simulink model "MotDynamic"  (R2020a)
settings: Solver=VariableStepAuto  StartTime=0.0  StopTime=inf  RelTol=1e-3  EnableMultiTasking=on
model workspace (MAT data in the model file):
  EV_current = 200
  EV_motion = [20 4 0.8]
  EV_sf = 2000
  Fs = 0
  Fv = 0.0025
  Jcomp = 0.0227
  Ki = 1.25663706144
  Kisa = 346.6583
  Kp_d = 0.648424723701
  Kp_q = 1.13097335529
  Ksa = 85.4316
  Ksf = 1996.2651
  Ld = 0.000516
  Ldq = [0.000516 0.0009]
  Lq = 0.0009
  Mechanical = [0.0227 0.0025 0]
  P = 4
  PolePairs = 4
  Rs = 0.001
  T_max = 307
  T_mtpa = [0 30.6210532811 61.5690748203 93.1444955648 125.603920089 159.154914294 193.959648015 230.142548009 267.798503723 307.000007318]
  ba = 3.4029
  id_mtpa = [0 -1.69646410405 -6.64649055035 -14.4836473325 -24.7304283732 -36.9068843148 -50.593409792 -65.4508356078 -81.216288034 -97.6899955843]
  idq0 = [0 0]
  idq_limits = [-97.6904029428 235.234863652 254.71328176]
  iq_mtpa = [0 28.2505847591 56.2113714662 83.6599409941 110.471636122 136.609736594 162.096742578 186.986339268 211.343844145 235.235032823]
  lambda_pm = 0.18
  mechanical = [0.0227 0.0025 0]
  omega_init = 0
  theta_init = 0
libraries: autolibmotorctrlr x1, autolibpmsminterior x1, autolibinverter x1
settings Model: ModifiedByFormat=The MathWorks, Inc.  SimulationMode=accelerator  PauseTimes=10  Creator=The MathWorks, Inc.  LastModifiedBy=The MathWorks, Inc.
settings SolverCC: DecoupledContinuousIntegration=on
settings DataIOCC: DSMLogging=off  ReturnWorkspaceOutputs=off
settings DebuggingCC: UnderspecifiedInitializationDetection=Classic  MergeDetectMultiDrivingBlocksExec=none  ArithmeticOperatorsInVariantConditions=warning
settings ModelReferenceCC: PropagateSignalLabelsOutOfModel=off
settings SFSimCC: SimUseLocalCustomCode=off  CustomCodeUndefinedFunction=UseInterfaceOnly
settings RTWCC: RTWUseLocalCustomCode=off
settings CodeAppCC: StateflowObjectComments=on
settings GRTTargetCC: TargetLangStandard=C89/C90 (ANSI)
settings ConfigComp: CovMetricSettings=dsw  CovHtmlReporting=on  CovSaveCumulativeToWorkspaceVar=on  CovSaveSingleToWorkspaceVar=on  CovShowResultsExplorer=off  CovExternalEMLEnable=off
settings SimscapeCC: SimscapeNormalizeSystem=off  SimscapeNominalValues={1, 'bar'; 1, 'cm^3/s'; 1, 'bar*kg/s'; 1, 'kJ/kg'; 1, 'kW'; }

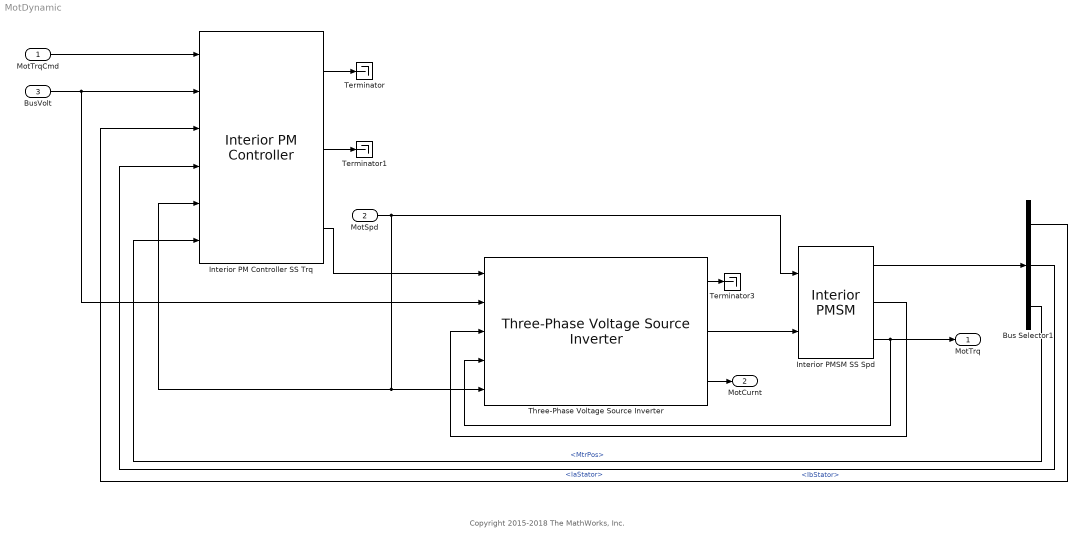
== system MotDynamic ==
  note: Copyright 2015-2018 The MathWorks, Inc.
  MotTrqCmd : Inport
  MotSpd : Inport  Port=2
  BusVolt : Inport  Port=3
  Bus Selector1 : BusSelector  OutputSignals=IaStator,IbStator,MtrPos
  Interior PM Controller SS Trq : autolibmotorctrlr/Interior PM Controller  control_type=Torque Control  Rs=Rs  Ld=Ld  Lq=Lq  lambda_pm=lambda_pm  PolePairs=PolePairs  Mechanical=Mechanical  T_max=T_max  bp=10  T_mtpa=T_mtpa  id_mtpa=id_mtpa  iq_mtpa=iq_mtpa  idq_limits=idq_limits  EV_current=EV_current  Tst=5e-5  Kp_d=Kp_d  Kp_q=Kp_q  Ki=Ki  EV_motion=EV_motion  EV_sf=EV_sf  ba=ba  Ksa=Ksa  Kisa=Kisa  Ksf=Ksf  Jcomp=Jcomp  Fv=Fv  Fs=Fs  param_loss=Single efficiency measurement  eff=98  w_loss_bp=[0 200 400 600 800 1000]  T_loss_bp=[0 25 50 75 100]  losses_table=[100 100 100 100 100;100 150 200 250 300;100 200 300 400 500;100 250 400 550 700;100 300 500 700 900;100 350 600 850 1100]  w_eff_bp=[200 400 600 800 1000]  T_eff_bp=[25 50 75 100]  efficiency_table=[96.2 98.1 98.7 99;98.1 99 99.4 99.5;98.7 99.4 99.6 99.7;99 99.5 99.7 99.8;99.2 99.6 99.7 99.8]  x_w_bp=[-1000 -800 -600 -400 -200 200 400 600 800 1000]  x_T_bp=[-100 -75 -50 -25 25 50 75 100]  x_losses_mat=[200.400801603196 225.67703109328 200.803212851408 201.612903225806 199.999999999997 200 225 200;160.320641282556 180.541624874624 201.005025125625 202.020202020203 200 200 180 160;180.541624874624 180.722891566267 181.086519114686 197.568389057748 194.999999999999 179.999999999997 180 180;201.005025125625 181.086519114686 202.020202020203 193.67991845056 190 200 179.999999999997 200;202.020202020203 197.568389057748 193.67991845056 197.505197505197 190 190 194.999999999999 200;200 194.999999999999 190 190 197.505197505197 193.67991845056 197.568389057748 202.020202020203;200 179.999999999997 200 190 193.67991845056 202.020202020203 181.086519114686 201.005025125625;180 180 179.999999999997 194.999999999999 197.568389057748 181.086519114686 180.722891566267 180.541624874624;160 180 200 200 202.020202020203 201.005025125625 180.541624874624 160.320641282556;200 225 200 199.999999999997 201.612903225806 200.803212851408 225.67703109328 200.400801603196]  Tsm=5e-4
      settings: SourceProductBaseCode=PW
  Interior PMSM SS Spd : autolibpmsminterior/Interior PMSM  port_config=Speed  sim_type=Continuous  Ts=0.001  P=P  Rs=Rs  Ldq=Ldq  KConstText=Permanent flux linkage constant (lambda_pm):  lambda_pm=lambda_pm  Ke=159.9771  mechanical=mechanical  idq0=idq0  theta_init=theta_init  omega_init=omega_init  KConst=lambda_pm  lambda_pm_calc=lambda_pm  Kt=1.323  RefBlkName='autolibpmsminterior/Interior PMSM'  aMode=1
      settings: SourceProductBaseCode=PW,MT,VE,VP
  Terminator : Terminator
  Terminator1 : Terminator
  Terminator3 : Terminator
  Three-Phase Voltage Source Inverter : autolibinverter/Three-Phase Voltage Source Inverter  InvrtrTmpInpEnbl=off  enable_hdl=off  model_type=Commanded phase voltage  fs=5000  w_eff_bp=[-1000 -500 0 500 1000]  n1=128  T_eff_bp=[-200 -100 0 100 200]  Temp_eff_bp=[213.15 293.15 373.15]  n2=128  ploss_table=0.98*ones(5,5)  ploss_table_3d=cat(3,0.95*[1 0.999 0.989 0.997 0.996;0.995 0.994 0.993 0.992 0.991;0.990 0.989 0.988 0.987 0.986;0.985 0.984 0.983 0.982 0.981;0.980 0.979 0.978 0.977 0.976],[1 0.999 0.989 0.997 0.996;0.995 0.994 0.993 0.992 0.991;0.990 0.989 0.988 0.987 0.986;0.985 0.984 0.983 0.982 0.981;0.980 0.979 0.978 0.977 0.976],0.92*[1 0.999 0.989 0.997 0.996;0.995 0.994 0.993 0.992 0.991;0.990 0.989 0.988 0.987 0.986;0.985 0.984 0.983 0.982 0.981;0.980 0.979 0.978 0.977 0.976])  preExtrapFlag=off  u1max=1000  u1min=-1000  u2max=200  u2min=-200  intPrec=23  RefBlkName='autolibmappedmotor/Mapped Motor'  CalLossMapData={}  CalLossWithTempMapData={}
      settings: SourceProductBaseCode=PW,MT,VE,VP
  MotTrq : Outport  VectorParamsAs1DForOutWhenUnconnected=off
  MotCurnt : Outport  Port=2  VectorParamsAs1DForOutWhenUnconnected=off
  wires:
  Interior PM Controller SS Trq/2 -> Terminator1/1
  Three-Phase Voltage Source Inverter/2 -> Interior PMSM SS Spd/2
  Three-Phase Voltage Source Inverter/3 -> MotCurnt/1
  Interior PMSM SS Spd/2 -> Three-Phase Voltage Source Inverter/3
  Three-Phase Voltage Source Inverter/1 -> Terminator3/1
  Bus Selector1/1 -> Interior PM Controller SS Trq/3  "<IaStator>"
  Interior PMSM SS Spd/1 -> Bus Selector1/1
  Bus Selector1/3 -> Interior PM Controller SS Trq/6  "<MtrPos>"
  MotSpd/1 -> Interior PMSM SS Spd/1, Interior PM Controller SS Trq/5, Three-Phase Voltage Source Inverter/5
  Interior PM Controller SS Trq/1 -> Terminator/1
  Interior PM Controller SS Trq/3 -> Three-Phase Voltage Source Inverter/1
  MotTrqCmd/1 -> Interior PM Controller SS Trq/1
  BusVolt/1 -> Interior PM Controller SS Trq/2, Three-Phase Voltage Source Inverter/2
  Bus Selector1/2 -> Interior PM Controller SS Trq/4  "<IbStator>"
  Interior PMSM SS Spd/3 -> Three-Phase Voltage Source Inverter/4, MotTrq/1
